simulink model "v0_sym"  (R2023b)
settings: Solver=VariableStepAuto  StartTime=0.0  StopTime=1  RelTol=1e-3
values from neighbouring files (symbols this model uses):
  K = [-1651800 2200]    [WP1.m]    (also in dynamic_performance.m)
  kr = -1636751    [WP1.m]    (also in dynamic_performance.m)
settings Model: Creator=kiraa  LastModifiedBy=kiraa

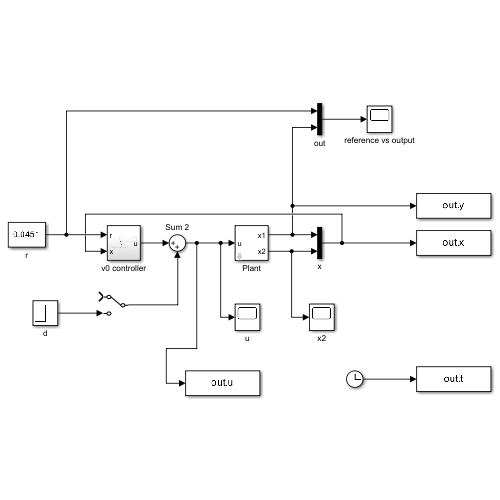
[thumbnail: Simulink's stored preview of the top-level diagram]
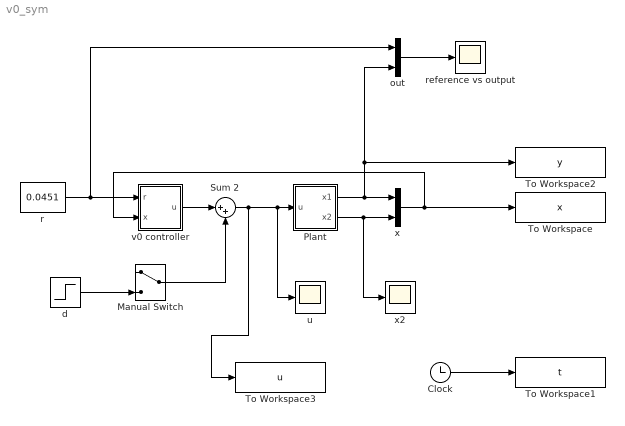
== system v0_sym ==
  Clock : Clock
  Manual Switch : ManualSwitch
  Plant : Subsystem  mask{x1_0=0.001, x2_0=0.01}
      mask prompts: x1_0 "x1(0) [g/l]"; x2_0 "x2(0) [min^-1]"
  Sum 2 : Sum  Inputs=|++
  To Workspace : ToWorkspace  VariableName=x  SampleTime=-1
  To Workspace1 : ToWorkspace  VariableName=t  SaveFormat=Timeseries  SampleTime=-1
  To Workspace2 : ToWorkspace  VariableName=y  SampleTime=-1
  To Workspace3 : ToWorkspace  VariableName=u  SampleTime=-1
  d : Step  Time=0.5  After=20000  SampleTime=0
  out : Mux  Inputs=2
  r : Constant  Value=0.0451
  reference vs output : Scope
  u : Scope
  v0 controller : Subsystem
  x : Mux  Inputs=2
  x2 : Scope
  wires:
  Clock/1 -> To Workspace1/1
  r/1 -> out/1, v0 controller/1(r)
  x/1 -> v0 controller/2(x), To Workspace/1
  out/1 -> reference vs output/1
  Plant/1(x1) -> out/2, To Workspace2/1, x/1
  Plant/2(x2) -> x2/1, x/2
  Sum 2/1 -> To Workspace3/1, Plant/1(u), u/1
  d/1 -> Manual Switch/2
  Manual Switch/1 -> Sum 2/2
  v0 controller/1(u) -> Sum 2/1

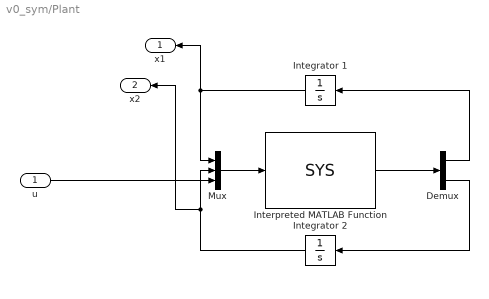
== system v0_sym/Plant ==
  u : Inport
  Demux : Demux  Outputs=2
  Integrator 1 : Integrator  InitialCondition=x1_0
  Integrator 2 : Integrator  InitialCondition=x2_0
  Interpreted MATLAB Function : MATLABFcn  MATLABFcn=SYS  OutputDimensions=2
  Mux : Mux  Inputs=3
  x1 : Outport
  x2 : Outport  Port=2
  wires:
  Integrator 1/1 -> x1/1, Mux/1
  Demux/1 -> Integrator 1/1
  Mux/1 -> Interpreted MATLAB Function/1
  Integrator 2/1 -> x2/1, Mux/2
  Interpreted MATLAB Function/1 -> Demux/1
  Demux/2 -> Integrator 2/1
  u/1 -> Mux/3

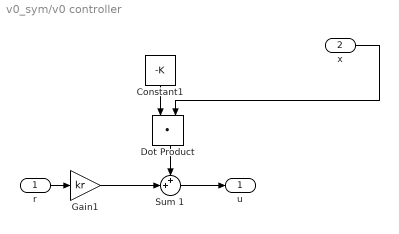
== system v0_sym/v0 controller ==
  r : Inport
  x : Inport  Port=2
  Constant1 : Constant  Value=-K
  Dot Product : DotProduct  OutDataTypeStr=Inherit: Inherit via internal rule
  Gain1 : Gain  Gain=kr
  Sum 1 : Sum  Inputs=++|
  u : Outport
  wires:
  Dot Product/1 -> Sum 1/1
  x/1 -> Dot Product/2
  r/1 -> Gain1/1
  Constant1/1 -> Dot Product/1
  Gain1/1 -> Sum 1/2
  Sum 1/1 -> u/1
